simulink model "AFCS_2"  (R2016a)
settings: Solver=VariableStepAuto  StartTime=0.0  StopTime=10.0  RelTol=1e-3
values from neighbouring files (symbols this model uses):
  A = [ ... (first row only)    [AFCS.m]
  B = [ ... (first row only)    [AFCS.m]
  collective = 0    [AFCS.m]
  H1 = inv(B'*B)*B'*B1d    [AFCS.m]
  K1 = inv((B'*B))*B'*(A-A1d)    [AFCS.m]
  lateral = 0    [AFCS.m]
  longtudinal = 1    [AFCS.m]
  pedal = 0    [AFCS.m]
settings Model: Creator=Administrator  LastModifiedBy=Administrator

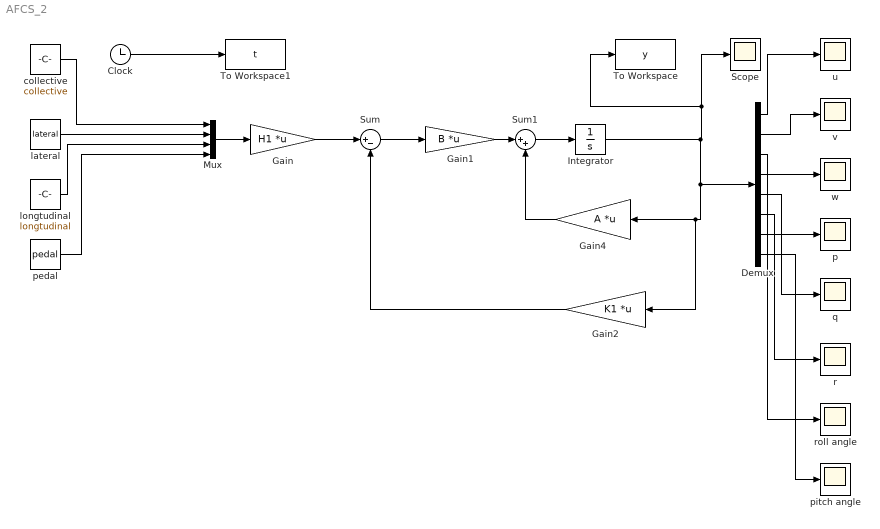
== system AFCS_2 ==
  Clock : Clock
  Demux : Demux  Outputs=8
  Gain : Gain  Gain=H1  Multiplication=Matrix(K*u)
  Gain1 : Gain  Gain=B  Multiplication=Matrix(K*u)
  Gain2 : Gain  Gain=K1  Multiplication=Matrix(K*u)
  Gain4 : Gain  Gain=A  Multiplication=Matrix(K*u)
  Integrator : Integrator
  Mux : Mux
  Scope : Scope
  Sum : Sum  Inputs=|+-
  Sum1 : Sum  Inputs=|++
  To Workspace : ToWorkspace  VariableName=y  SampleTime=-1
  To Workspace1 : ToWorkspace  VariableName=t  SampleTime=-1
  collective : Constant  Value=collective
  lateral : Constant  Value=lateral
  longtudinal : Constant  Value=longtudinal
  p : Scope
  pedal : Constant  Value=pedal
  pitch angle : Scope
  q : Scope
  r : Scope
  roll angle : Scope
  u : Scope
  v : Scope
  w : Scope
  wires:
  collective/1 -> Mux/1
  lateral/1 -> Mux/2
  longtudinal/1 -> Mux/3
  pedal/1 -> Mux/4
  Mux/1 -> Gain/1
  Gain/1 -> Sum/1
  Sum/1 -> Gain1/1
  Sum1/1 -> Integrator/1
  Integrator/1 -> Gain2/1, Gain4/1, Demux/1, Scope/1, To Workspace/1
  Gain4/1 -> Sum1/2
  Gain2/1 -> Sum/2
  Gain1/1 -> Sum1/1
  Demux/1 -> u/1
  Demux/2 -> v/1
  Demux/3 -> w/1
  Demux/4 -> p/1
  Demux/5 -> q/1
  Demux/6 -> r/1
  Demux/7 -> roll angle/1
  Demux/8 -> pitch angle/1
  Clock/1 -> To Workspace1/1
